simulink model "NPC_MPC_rtiFPGASeparationFile"  (R2018b)
settings: Solver=FixedStepAuto  StartTime=0.0  StopTime=Inf  FixedStep=10e-6  RelTol=1e-3
PostLoadFcn:
  | , if any(exist('dsrtsu_mdlpostloadfcn', 'file') ~= 0), dsrtsu_mdlpostloadfcn('Execute', bdroot); end,
values from neighbouring files (symbols this model uses):
  Amplitude = 1    [params.m]
  L = 10e-3    (= 0.01)    [params.m]
  R = 7.5    [params.m]
  S = [-1 -1 -1 ... (first row only)    [params.m]
undefined symbols (not defined in the file or in its folder): T
libraries: xbsIndex_r4 x282, rti1202lib_adc_class1 x3, rtiproclib x3, simulink x1, rtifpgainterfacelib x1
(part 6 of 6)

== system NPC_MPC_rtiFPGASeparationFile/RTI Data/RTI Data Store/RTI Data Store/RTI Data Store/RTI Data Store ==

== matlab function NPC_MPC_rtiFPGASeparationFile/Subsystem/MATLAB Function ==
  data: iref input; i input; state output; S parameter; R parameter; L parameter; T parameter; Vdc input
function state = fcn(iref, i, S, R, L, T, Vdc)
kopt = 1;
Jmin = inf;
for k=1:27
    vnpc = (Vdc/2).*S(k,:)';
    v = [2/3 -1/3 -1/3; -1/3 2/3 -1/3; -1/3 -1/3 2/3]*vnpc;
    ikk = (1-R*T/L)*i +(T/L)*v;
    ei = iref-ikk;
    J = ei'*ei;
    if(J<Jmin)
        Jmin = J;
        kopt = k;
    end
end
state = kopt;
